simulink library "inputs"  (Simulink 3.00)
values from neighbouring files (symbols this model uses):
  tx = t-to    [ag1.m]

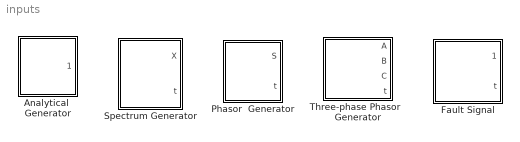
== system inputs ==
  Analytical  Generator : Subsystem  mask(Analytical Generator){y=10*cos(2*pi*60*tx), to=1/60}
      mask prompts: y "Generated function"; to "Start-up time [sec]"
      mask help: Generates any signal by providing the equation describing the output value. The time variable must be named tx. The start-up time must be specified.
      mask init:
      | t = 0:0.001:0.1;
      | 
      | for i = 1:length(t)
      |   if t(i) < to
      |     x(i) = 0;
      |   else
      |     tx = t(i) - to;
      |     x(i) =  eval(y);
      |   end
      | end
      mask Help: web(['file:///' which('agdoc.html')]);
      mask Display: plot(t,x);
  Fault Signal : Subsystem  mask(Fault Signal Generator){pre_fault=[10 45], post_fault=[2 90], fr_dc=[60 1.25/60 0.0004], oscA=[1.0 0.8 0.9], oscf=[1000 3000 8000], oscT=[0.050 0.030 0.060]}
      mask prompts: pre_fault "Pre-fault amplitude and phase [degrees]"; post_fault "Fault amplitude and phase [degrees]"; fr_dc "Frequency [Hz], fault time and DC time constant"; oscA "Amplitudes of the oscillatory components"; oscf "Frequencies of the oscillatory components"; oscT "Time constants of the oscillatory components"
      mask help: Generates a signal which evolves from a given pre-fault phasor to a given post-fault phasor. A limited number of decaying high frequency components are included. The d.c. component is also included. The start-up time may be specified.
      mask init:
      | tx=0:4*fr_dc(2)/100:4*fr_dc(2);
      | out(1:26)=pre_fault(1)*cos(2*pi*fr_dc(1)*tx(1:26)+pre_fault(2)*pi/180);
      | a=out(26);
      | out(26:101)=post_fault(1)*cos(2*pi*fr_dc(1)*tx(26:101)+post_fault(2)*pi/180);
      | Adc=a-out(26);
      | for  k = 26:101
      |       wt=2.*pi.*(tx(k)-fr_dc(2)).*oscf;
      |       osc(k)=sum(oscA.*exp(-(tx(k)-fr_dc(2))./oscT).*sin(wt));
      | end
      | out(26:101)=out(26:101)+Adc*exp(-(tx(26:101)-fr_dc(2))/fr_dc(3))+osc(26:101);
      mask Help: web(['file:///' which('fsgdoc.html')]);
      mask Display: plot(tx,out);
  Phasor  Generator : Subsystem  mask(Phasor Generator){phase1=[10 45], f=60, to=1.25/60}
      mask prompts: phase1 "Phasor   [amplitude, phase in degree]"; f "Frequency [Hz]"; to "Start time [sec]"
      mask help: Generates a pure sinusoid waveform. The parameters of the output signal that have to be specified include amplitude, phase and frequency as well as the start-up time..
      mask init:
      | xo  = 0;
      | yo  = 0;
      | Amax = abs(phase1(1));
      | x1 = phase1(1)*cos(phase1(2)*pi/180);
      | y1 = phase1(1)*sin(phase1(2)*pi/180);
      mask Help: web(['file:///' which('pgdoc.html')]);
      mask Display:
      | plot([0 0], [ 0  Amax/8]);
      | plot([0 0], [3*Amax/8 5*Amax/8]);
      | plot([0 0], [7*Amax/8 Amax]);
      | plot([0 0], [0 -Amax/8]);
      | plot([0 0], [-3*Amax/8 -5*Amax/8]);
      | plot([0 0], [-7*Amax/8 -Amax]);
      | 
      | plot([ 0  Amax/8], [0 0]);
      | plot([3*Amax/8 5*Amax/8], [0 0]);
      | plot([7*Amax/8 Amax], [0 0]);
      | plot([0 -Amax/8], [0 0]);
      | plot([-3*Amax/8 -5*Amax/8], [ 0 0]);
      | plot([-7*Amax/8 -Amax], [0 0]);
      | 
      | plot([xo x1], [yo y1]);
  Spectrum Generator : Subsystem  mask(Spectrum Generator){f=60, m=[0 1/3 1 2 5], A=[0.1 0.2 1 0.25 0.15], ph=[0 0 0 30 45], to=1/60}
      mask prompts: f "Fundamental frequency [Hz]"; m "Frequency multipliers"; A "Amplitudes"; ph "Phases [deg]"; to "Start-up time [sec]"
      mask help: Generates a signal composed from the limited number of harmonics and sub-harmonics including the d.c. component. For each signal component, the amplitude, phase and harmonic order are the parameters. The start-up time may be specified. The frequency for each component expressed as multiple of the fundamental frequency is specyfied in the frequency multipliers array.
      mask init:
      | for i = 1:3:3*length(A)
      |    x(i)   = i;
      |    x(i+1) = i;
      |    x(i+2) = i;
      | end
      | 
      | W = zeros(length(A),3);
      | W(:,2) = A';
      | W = W';
      | for i = 1:3*length(A)
      |    y(i) = W(i);
      | end
      mask Help: web(['file:///' which('scdoc.html')]);
      mask Display: plot(x,y);
  Three-phase Phasor   Generator : Subsystem  mask(Three-phase phasor generator){phase_type=Phase quantities-symmetrical, phase1=[10 45], phase2=[0 150], phase3=[0 -50], f=60, to=0}
      mask prompts: phase_type "Three-phase phasors"; phase1 "Phasor (A or 0);  [amplitude, phase in degree]"; phase2 "Phasor (B or 1);  [amplitude, phase in degree]"; phase3 "Phasor (C or 2);  [amplitude, phase in degree]"; f "Frequency [Hz]"; to "Start-up time [sec]"
      mask help: Generates three pure sinusoid waveforms. The parameters of the output signals to be specified include amplitude and phase for each phasor as well as the frequency and the start-up time. The phasors may be set either as phase or symmetrical component values.
      mask init:
      | TPG2
      mask Help: web(['file:///' which('tpgdoc.html')]);
      mask StyleString: popup(Phase quantities-symmetrical|Phase quantities-unsymmetrical|Symmetrical components),edit,edit,edit,edit,edit
      mask Display:
      | plot([0 0], [ 0  Amax/8]);
      | plot([0 0], [3*Amax/8 5*Amax/8]);
      | plot([0 0], [7*Amax/8 Amax]);
      | plot([0 0], [0 -Amax/8]);
      | plot([0 0], [-3*Amax/8 -5*Amax/8]);
      | plot([0 0], [-7*Amax/8 -Amax]);
      | 
      | plot([ 0  Amax/8], [0 0]);
      | plot([3*Amax/8 5*Amax/8], [0 0]);
      | plot([7*Amax/8 Amax], [0 0]);
      | plot([0 -Amax/8], [0 0]);
      | plot([-3*Amax/8 -5*Amax/8], [ 0 0]);
      | plot([-7*Amax/8 -Amax], [0 0]);
      | 
      | plot([xo x1], [yo y1], [xo x2], [yo y2], [xo x3], [yo y3]);

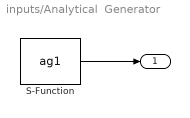
== system inputs/Analytical  Generator ==
  S-Function : S-Function  FunctionName=ag1  Parameters=y,to  PortCounts=[]  SFunctionModules=''
  "              " : Outport  Port=1
  wires:
  S-Function/1 -> "              "/1

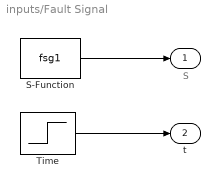
== system inputs/Fault Signal ==
  note: S
  S-Function : S-Function  FunctionName=fsg1  Parameters=pre_fault,post_fault,fr_dc,oscA,oscf,oscT  PortCounts=[]  SFunctionModules=''
  Time : Step  Time=fr_dc(2)  Before=0  After=1  SampleTime=-1
  " " : Outport  Port=1  InitialOutput=0
  t : Outport  Port=2  InitialOutput=0
  wires:
  Time/1 -> t/1
  S-Function/1 -> " "/1

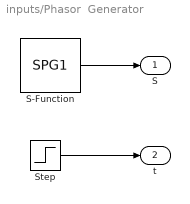
== system inputs/Phasor  Generator ==
  S-Function : S-Function  FunctionName=SPG1  Parameters=phase1,f,to  PortCounts=[]  SFunctionModules=''
  Step : Step  Time=to  Before=0  After=1  SampleTime=-1
  S : Outport  Port=1
  t : Outport  Port=2
  wires:
  Step/1 -> t/1
  S-Function/1 -> S/1

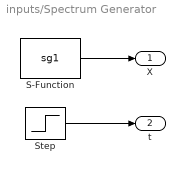
== system inputs/Spectrum Generator ==
  S-Function : S-Function  FunctionName=sg1  Parameters=f,m,A,ph,to  PortCounts=[]  SFunctionModules=''
  Step : Step  Time=to  Before=0  After=1  SampleTime=-1
  X : Outport  Port=1
  t : Outport  Port=2
  wires:
  S-Function/1 -> X/1
  Step/1 -> t/1

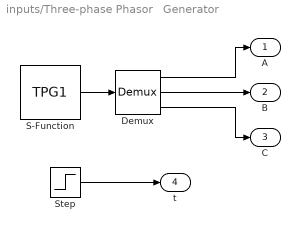
== system inputs/Three-phase Phasor   Generator ==
  Demux : Demux  Outputs=3
  S-Function : S-Function  FunctionName=TPG1  Parameters=phase_type,phase1,phase2,phase3,f,to  PortCounts=[]  SFunctionModules=''
  Step : Step  Time=to  Before=0  After=1  SampleTime=-1
  A : Outport  Port=1
  B : Outport  Port=2
  C : Outport  Port=3
  t : Outport  Port=4
  wires:
  Step/1 -> t/1
  S-Function/1 -> Demux/1
  Demux/1 -> A/1
  Demux/3 -> C/1
  Demux/2 -> B/1
